simulink model "Control_Loop4_2Model"  (R2013b)
settings: Solver=ode45  StartTime=0.0  StopTime=200  RelTol=1e-3
libraries: commutil2 x756, xpclib x100, etargetslib x98, dspnetwork x98, powerlib_meascontrol x24, commcrc2 x14, dspadpt3 x4, simulink_extras x4, dspmtrx3 x4, simulink x1
(part 7 of 7)

== system Control_Loop4_2Model/GISOO-Simulation Environment/SkyMote8/Subsystem ==
  SerialData : Inport
  AM Packet type : Constant  Value=PacketType  OutDataTypeStr=double
  Bit to Integer Converter{,1..27} (28 alike) : commutil2/Bit to Integer Converter  nbits=8  bitOrder=MSB first  signedOutputValues=Unsigned  outDtype=Inherit via internal rule  outDtypeSigned=Inherit via internal rule
  Constant25 : Constant  Value=72  OutDataTypeStr=double
  Constant26 : Constant  Value=0  OutDataTypeStr=double
  Constant{27..30} (4 alike) : Constant  Value=255  OutDataTypeStr=double
  Constant31 : Constant  Value=16  OutDataTypeStr=double
  Constant32 : Constant  Value=137  OutDataTypeStr=double
  Demux1 : Demux  Outputs=28
  Demux2 : Demux  Outputs=16
  FrameByteEnd : Constant  Value=126  OutDataTypeStr=uint8
  FrameByteStart : Constant  Value=126  OutDataTypeStr=uint8
  Framing byte : Constant  Value=68  OutDataTypeStr=uint8
  General CRC Generator1 : commcrc2/General CRC Generator  genPoly=[1 0 0 0 1 0 0 0 0 0 0 1 0 0 0 0 1]  iniStates=0  directMethod=off  reflectInputBytes=off  reflectChecksums=off  finalXOR=0  numChecksums=1
  Integer to Bit Converter{,1..25} (26 alike) : commutil2/Integer to Bit Converter  nbits=8  signedInputValues=Unsigned  bitOrder=MSB first  outDtype=boolean
  Mux1 : Mux  Inputs=26
  Mux2 : Mux  Inputs=30
  SerialFrame : Outport
  wires:
  Bit to Integer Converter27/1 -> Mux2/3
  Demux1/28 -> Bit to Integer Converter27/1
  FrameByteStart/1 -> Mux2/30
  Bit to Integer Converter26/1 -> Mux2/2
  Demux1/27 -> Bit to Integer Converter26/1
  Demux1/15 -> Bit to Integer Converter18/1
  Demux1/14 -> Bit to Integer Converter13/1
  Demux1/6 -> Bit to Integer Converter5/1
  Demux1/16 -> Bit to Integer Converter19/1
  Demux1/25 -> Bit to Integer Converter22/1
  Demux1/17 -> Bit to Integer Converter14/1
  Demux1/18 -> Bit to Integer Converter15/1
  Demux1/26 -> Bit to Integer Converter23/1
  Demux1/22 -> Bit to Integer Converter25/1
  Demux1/23 -> Bit to Integer Converter20/1
  Demux1/20 -> Bit to Integer Converter17/1
  Demux1/19 -> Bit to Integer Converter16/1
  Demux1/5 -> Bit to Integer Converter4/1
  Demux1/21 -> Bit to Integer Converter24/1
  Demux1/4 -> Bit to Integer Converter3/1
  Demux1/24 -> Bit to Integer Converter21/1
  Constant31/1 -> Integer to Bit Converter7/1
  Integer to Bit Converter19/1 -> Mux1/20
  Integer to Bit Converter20/1 -> Mux1/21
  Integer to Bit Converter9/1 -> Mux1/10
  Integer to Bit Converter18/1 -> Mux1/19
  Demux1/12 -> Bit to Integer Converter11/1
  Mux2/1 -> SerialFrame/1
  Integer to Bit Converter12/1 -> Mux1/13
  Demux2/9 -> Integer to Bit Converter18/1
  Demux1/7 -> Bit to Integer Converter6/1
  Demux1/13 -> Bit to Integer Converter12/1
  Demux1/9 -> Bit to Integer Converter8/1
  Demux1/1 -> Bit to Integer Converter/1
  Demux2/11 -> Integer to Bit Converter20/1
  Demux1/11 -> Bit to Integer Converter10/1
  AM Packet type/1 -> Integer to Bit Converter9/1
  FrameByteEnd/1 -> Mux2/1
  Integer to Bit Converter22/1 -> Mux1/23
  Integer to Bit Converter21/1 -> Mux1/22
  Integer to Bit Converter25/1 -> Mux1/26
  Constant32/1 -> Integer to Bit Converter8/1
  Integer to Bit Converter8/1 -> Mux1/9
  General CRC Generator1/1 -> Demux1/1
  Integer to Bit Converter7/1 -> Mux1/8
  Demux1/3 -> Bit to Integer Converter2/1
  Integer to Bit Converter2/1 -> Mux1/3
  Integer to Bit Converter3/1 -> Mux1/4
  Constant28/1 -> Integer to Bit Converter4/1
  Integer to Bit Converter4/1 -> Mux1/5
  Constant27/1 -> Integer to Bit Converter3/1
  Constant26/1 -> Integer to Bit Converter2/1
  Constant29/1 -> Integer to Bit Converter5/1
  Integer to Bit Converter1/1 -> Mux1/2
  Integer to Bit Converter5/1 -> Mux1/6
  Demux2/14 -> Integer to Bit Converter23/1
  Demux2/16 -> Integer to Bit Converter25/1
  Mux1/1 -> General CRC Generator1/1
  Framing byte/1 -> Integer to Bit Converter/1
  Demux2/15 -> Integer to Bit Converter24/1
  Demux2/13 -> Integer to Bit Converter22/1
  Integer to Bit Converter/1 -> Mux1/1
  Demux2/12 -> Integer to Bit Converter21/1
  Constant25/1 -> Integer to Bit Converter1/1
  Demux2/8 -> Integer to Bit Converter17/1
  Integer to Bit Converter10/1 -> Mux1/11
  Demux2/10 -> Integer to Bit Converter19/1
  Integer to Bit Converter6/1 -> Mux1/7
  Demux1/2 -> Bit to Integer Converter1/1
  Integer to Bit Converter16/1 -> Mux1/17
  Integer to Bit Converter15/1 -> Mux1/16
  Integer to Bit Converter17/1 -> Mux1/18
  Integer to Bit Converter13/1 -> Mux1/14
  Demux1/8 -> Bit to Integer Converter7/1
  Demux1/10 -> Bit to Integer Converter9/1
  Constant30/1 -> Integer to Bit Converter6/1
  Integer to Bit Converter11/1 -> Mux1/12
  Integer to Bit Converter23/1 -> Mux1/24
  Integer to Bit Converter24/1 -> Mux1/25
  Integer to Bit Converter14/1 -> Mux1/15
  Demux2/6 -> Integer to Bit Converter15/1
  Demux2/5 -> Integer to Bit Converter14/1
  Bit to Integer Converter22/1 -> Mux2/5
  SerialData/1 -> Demux2/1
  Bit to Integer Converter21/1 -> Mux2/6
  Demux2/2 -> Integer to Bit Converter11/1
  Demux2/1 -> Integer to Bit Converter10/1
  Bit to Integer Converter17/1 -> Mux2/10
  Bit to Integer Converter20/1 -> Mux2/7
  Bit to Integer Converter/1 -> Mux2/29
  Bit to Integer Converter9/1 -> Mux2/20
  Bit to Integer Converter7/1 -> Mux2/22
  Bit to Integer Converter11/1 -> Mux2/18
  Bit to Integer Converter4/1 -> Mux2/25
  Bit to Integer Converter1/1 -> Mux2/28
  Bit to Integer Converter6/1 -> Mux2/23
  Bit to Integer Converter10/1 -> Mux2/19
  Bit to Integer Converter25/1 -> Mux2/8
  Bit to Integer Converter15/1 -> Mux2/12
  Bit to Integer Converter13/1 -> Mux2/16
  Bit to Integer Converter16/1 -> Mux2/11
  Bit to Integer Converter2/1 -> Mux2/27
  Bit to Integer Converter5/1 -> Mux2/24
  Demux2/7 -> Integer to Bit Converter16/1
  Bit to Integer Converter14/1 -> Mux2/13
  Bit to Integer Converter19/1 -> Mux2/14
  Bit to Integer Converter12/1 -> Mux2/17
  Bit to Integer Converter18/1 -> Mux2/15
  Demux2/3 -> Integer to Bit Converter12/1
  Bit to Integer Converter8/1 -> Mux2/21
  Bit to Integer Converter24/1 -> Mux2/9
  Demux2/4 -> Integer to Bit Converter13/1
  Bit to Integer Converter3/1 -> Mux2/26
  Bit to Integer Converter23/1 -> Mux2/4

== system Control_Loop4_2Model/GISOO-Simulation Environment/SkyMote8/Triggered Subsystem ==
  In2 : Inport
  Trigger : TriggerPort
  Byte Reversal1 : etargetslib/Byte Reversal  numInp=1
  Data Type Conversion1 : DataTypeConversion  OutDataTypeStr=uint32
  Pack : xpclib/UDP/Pack  datatypes={'uint32'}  byteAlign=1
  UDP Send : dspnetwork/UDP Send  remoteURL='127.0.0.1'  remotePort=18000+moteID  localURL='0.0.0.0'  localPortSource=Automatically determine  localPort=-1  sampletime=-1  separateLengthPort=0
  wires:
  Data Type Conversion1/1 -> Byte Reversal1/1
  Byte Reversal1/1 -> Pack/1
  Pack/1 -> UDP Send/1
  In2/1 -> Data Type Conversion1/1

== system Control_Loop4_2Model/GISOO-Simulation Environment/SkyMote8/Triggered Subsystem1 ==
  In2 : Inport
  Trigger : TriggerPort
  Byte Reversal1 : etargetslib/Byte Reversal  numInp=1
  Data Type Conversion1 : DataTypeConversion  OutDataTypeStr=uint32
  Pack : xpclib/UDP/Pack  datatypes={'uint32'}  byteAlign=1
  UDP Send : dspnetwork/UDP Send  remoteURL='127.0.0.1'  remotePort=18000+moteID  localURL='0.0.0.0'  localPortSource=Automatically determine  localPort=-1  sampletime=-1  separateLengthPort=0
  wires:
  Byte Reversal1/1 -> Pack/1
  Data Type Conversion1/1 -> Byte Reversal1/1
  In2/1 -> Data Type Conversion1/1
  Pack/1 -> UDP Send/1

== system Control_Loop4_2Model/GISOO-Simulation Environment/SkyMote8/Triggered Subsystem2 ==
  In2 : Inport
  Trigger : TriggerPort
  Byte Reversal : etargetslib/Byte Reversal  numInp=1
  Data Type Conversion1 : DataTypeConversion  OutDataTypeStr=uint32
  Pack : xpclib/UDP/Pack  datatypes={'uint32'}  byteAlign=1
  UDP Send : dspnetwork/UDP Send  remoteURL='127.0.0.1'  remotePort=18000+moteID  localURL='0.0.0.0'  localPortSource=Automatically determine  localPort=-1  sampletime=-1  separateLengthPort=0
  Out1 : Outport
  wires:
  Byte Reversal/1 -> Pack/1
  Pack/1 -> UDP Send/1
  Data Type Conversion1/1 -> Byte Reversal/1, Out1/1
  In2/1 -> Data Type Conversion1/1

== system Control_Loop4_2Model/GISOO-Simulation Environment/SkyMote8/Triggered Subsystem3 ==
  In2 : Inport
  Trigger : TriggerPort
  Byte Reversal : etargetslib/Byte Reversal  numInp=1
  Data Type Conversion1 : DataTypeConversion  OutDataTypeStr=uint32
  Pack : xpclib/UDP/Pack  datatypes={'uint32'}  byteAlign=1
  UDP Send : dspnetwork/UDP Send  remoteURL='127.0.0.1'  remotePort=18000+moteID  localURL='0.0.0.0'  localPortSource=Automatically determine  localPort=-1  sampletime=-1  separateLengthPort=0
  Out1 : Outport
  wires:
  Byte Reversal/1 -> Pack/1
  In2/1 -> Data Type Conversion1/1
  Data Type Conversion1/1 -> Out1/1, Byte Reversal/1
  Pack/1 -> UDP Send/1

== system Control_Loop4_2Model/GISOO-Simulation Environment/SkyMote8/Triggered Subsystem4 ==
  RecivedSD : Inport
  Trigger : TriggerPort
  Byte Reversal : etargetslib/Byte Reversal  numInp=1
  Constant : Constant  Value=1111
  Data Type Conversion1 : DataTypeConversion  OutDataTypeStr=uint32
  Pack : xpclib/UDP/Pack  datatypes={'uint32'}  byteAlign=1
  UDP Send : dspnetwork/UDP Send  remoteURL='127.0.0.1'  remotePort=18000+moteID  localURL='0.0.0.0'  localPortSource=Automatically determine  localPort=-1  sampletime=-1  separateLengthPort=0
  SDToApplay : Outport
  wires:
  Data Type Conversion1/1 -> Byte Reversal/1
  Byte Reversal/1 -> Pack/1
  Constant/1 -> Data Type Conversion1/1
  RecivedSD/1 -> SDToApplay/1
  Pack/1 -> UDP Send/1

== system Control_Loop4_2Model/GISOO-Simulation Environment/SkyMote8/Triggered Subsystem5 ==
  SerialDataToSend : Inport
  Trigger : TriggerPort
  Byte Reversal : etargetslib/Byte Reversal  numInp=1
  Demux : Demux  Outputs=30
  Pack : xpclib/UDP/Pack  datatypes={'uint8','uint8','uint8','uint8','uint8','uint8','uint8','uint8','uint8','uint8','uint8','uint8','uint8','uint8','uint8','uint8','uint8','uint8','uint8','uint8','uint8','uint8','uint8','uint8','uint8','uint8','uint8','uint8','uint8','uint8'}  byteAlign=1
  UDP Send : dspnetwork/UDP Send  remoteURL='127.0.0.1'  remotePort=18000+moteID  localURL='0.0.0.0'  localPortSource=Automatically determine  localPort=-1  sampletime=-1  separateLengthPort=0
  wires:
  Pack/1 -> UDP Send/1
  Demux/1 -> Pack/1
  Demux/2 -> Pack/2
  Demux/3 -> Pack/3
  Demux/4 -> Pack/4
  Demux/5 -> Pack/5
  Demux/6 -> Pack/6
  Demux/7 -> Pack/7
  Demux/8 -> Pack/8
  Demux/9 -> Pack/9
  Demux/10 -> Pack/10
  Demux/11 -> Pack/11
  Demux/12 -> Pack/12
  Demux/13 -> Pack/13
  Demux/14 -> Pack/14
  Demux/15 -> Pack/15
  Demux/16 -> Pack/16
  Demux/17 -> Pack/17
  Demux/18 -> Pack/18
  Demux/19 -> Pack/19
  Demux/20 -> Pack/20
  Demux/21 -> Pack/21
  Demux/22 -> Pack/22
  Demux/23 -> Pack/23
  Demux/24 -> Pack/24
  Demux/25 -> Pack/25
  Demux/26 -> Pack/26
  Demux/27 -> Pack/27
  Demux/28 -> Pack/28
  Demux/29 -> Pack/29
  Demux/30 -> Pack/30
  SerialDataToSend/1 -> Byte Reversal/1
  Byte Reversal/1 -> Demux/1

== system Control_Loop4_2Model/GISOO-Simulation Environment/SkyMote9/ADC0 Sender ==
  In2 : Inport
  Trigger : TriggerPort
  Byte Reversal1 : etargetslib/Byte Reversal  numInp=1
  Data Type Conversion1 : DataTypeConversion  OutDataTypeStr=uint32
  Pack : xpclib/UDP/Pack  datatypes={'uint32'}  byteAlign=1
  UDP Send : dspnetwork/UDP Send  remoteURL='127.0.0.1'  remotePort=18000+moteID  localURL='0.0.0.0'  localPortSource=Automatically determine  localPort=-1  sampletime=-1  separateLengthPort=0
  wires:
  Data Type Conversion1/1 -> Byte Reversal1/1
  Byte Reversal1/1 -> Pack/1
  In2/1 -> Data Type Conversion1/1
  Pack/1 -> UDP Send/1

== system Control_Loop4_2Model/GISOO-Simulation Environment/SkyMote9/Subsystem ==
  SerialData : Inport
  AM Packet type : Constant  Value=PacketType  OutDataTypeStr=double
  Bit to Integer Converter{,1..27} (28 alike) : commutil2/Bit to Integer Converter  nbits=8  bitOrder=MSB first  signedOutputValues=Unsigned  outDtype=Inherit via internal rule  outDtypeSigned=Inherit via internal rule
  Constant25 : Constant  Value=72  OutDataTypeStr=double
  Constant26 : Constant  Value=0  OutDataTypeStr=double
  Constant{27..30} (4 alike) : Constant  Value=255  OutDataTypeStr=double
  Constant31 : Constant  Value=16  OutDataTypeStr=double
  Constant32 : Constant  Value=137  OutDataTypeStr=double
  Demux1 : Demux  Outputs=28
  Demux2 : Demux  Outputs=16
  FrameByteEnd : Constant  Value=126  OutDataTypeStr=uint8
  FrameByteStart : Constant  Value=126  OutDataTypeStr=uint8
  Framing byte : Constant  Value=68  OutDataTypeStr=uint8
  General CRC Generator1 : commcrc2/General CRC Generator  genPoly=[1 0 0 0 1 0 0 0 0 0 0 1 0 0 0 0 1]  iniStates=0  directMethod=off  reflectInputBytes=off  reflectChecksums=off  finalXOR=0  numChecksums=1
  Integer to Bit Converter{,1..25} (26 alike) : commutil2/Integer to Bit Converter  nbits=8  signedInputValues=Unsigned  bitOrder=MSB first  outDtype=boolean
  Mux1 : Mux  Inputs=26
  Mux2 : Mux  Inputs=30
  SerialFrame : Outport
  wires:
  Bit to Integer Converter27/1 -> Mux2/3
  Demux1/28 -> Bit to Integer Converter27/1
  FrameByteStart/1 -> Mux2/30
  Bit to Integer Converter26/1 -> Mux2/2
  Demux1/27 -> Bit to Integer Converter26/1
  Demux1/15 -> Bit to Integer Converter18/1
  Demux1/14 -> Bit to Integer Converter13/1
  Demux1/6 -> Bit to Integer Converter5/1
  Demux1/16 -> Bit to Integer Converter19/1
  Demux1/25 -> Bit to Integer Converter22/1
  Demux1/17 -> Bit to Integer Converter14/1
  Demux1/18 -> Bit to Integer Converter15/1
  Demux1/26 -> Bit to Integer Converter23/1
  Demux1/22 -> Bit to Integer Converter25/1
  Demux1/23 -> Bit to Integer Converter20/1
  Demux1/20 -> Bit to Integer Converter17/1
  Demux1/19 -> Bit to Integer Converter16/1
  Demux1/5 -> Bit to Integer Converter4/1
  Demux1/21 -> Bit to Integer Converter24/1
  Demux1/4 -> Bit to Integer Converter3/1
  Demux1/24 -> Bit to Integer Converter21/1
  Constant31/1 -> Integer to Bit Converter7/1
  Integer to Bit Converter19/1 -> Mux1/20
  Integer to Bit Converter20/1 -> Mux1/21
  Integer to Bit Converter9/1 -> Mux1/10
  Integer to Bit Converter18/1 -> Mux1/19
  Demux1/12 -> Bit to Integer Converter11/1
  Mux2/1 -> SerialFrame/1
  Integer to Bit Converter12/1 -> Mux1/13
  Demux2/9 -> Integer to Bit Converter18/1
  Demux1/7 -> Bit to Integer Converter6/1
  Demux1/13 -> Bit to Integer Converter12/1
  Demux1/9 -> Bit to Integer Converter8/1
  Demux1/1 -> Bit to Integer Converter/1
  Demux2/11 -> Integer to Bit Converter20/1
  Demux1/11 -> Bit to Integer Converter10/1
  AM Packet type/1 -> Integer to Bit Converter9/1
  FrameByteEnd/1 -> Mux2/1
  Integer to Bit Converter22/1 -> Mux1/23
  Integer to Bit Converter21/1 -> Mux1/22
  Integer to Bit Converter25/1 -> Mux1/26
  Constant32/1 -> Integer to Bit Converter8/1
  Integer to Bit Converter8/1 -> Mux1/9
  General CRC Generator1/1 -> Demux1/1
  Integer to Bit Converter7/1 -> Mux1/8
  Demux1/3 -> Bit to Integer Converter2/1
  Integer to Bit Converter2/1 -> Mux1/3
  Integer to Bit Converter3/1 -> Mux1/4
  Constant28/1 -> Integer to Bit Converter4/1
  Integer to Bit Converter4/1 -> Mux1/5
  Constant27/1 -> Integer to Bit Converter3/1
  Constant26/1 -> Integer to Bit Converter2/1
  Constant29/1 -> Integer to Bit Converter5/1
  Integer to Bit Converter1/1 -> Mux1/2
  Integer to Bit Converter5/1 -> Mux1/6
  Demux2/14 -> Integer to Bit Converter23/1
  Demux2/16 -> Integer to Bit Converter25/1
  Mux1/1 -> General CRC Generator1/1
  Framing byte/1 -> Integer to Bit Converter/1
  Demux2/15 -> Integer to Bit Converter24/1
  Demux2/13 -> Integer to Bit Converter22/1
  Integer to Bit Converter/1 -> Mux1/1
  Demux2/12 -> Integer to Bit Converter21/1
  Constant25/1 -> Integer to Bit Converter1/1
  Demux2/8 -> Integer to Bit Converter17/1
  Integer to Bit Converter10/1 -> Mux1/11
  Demux2/10 -> Integer to Bit Converter19/1
  Integer to Bit Converter6/1 -> Mux1/7
  Demux1/2 -> Bit to Integer Converter1/1
  Integer to Bit Converter16/1 -> Mux1/17
  Integer to Bit Converter15/1 -> Mux1/16
  Integer to Bit Converter17/1 -> Mux1/18
  Integer to Bit Converter13/1 -> Mux1/14
  Demux1/8 -> Bit to Integer Converter7/1
  Demux1/10 -> Bit to Integer Converter9/1
  Constant30/1 -> Integer to Bit Converter6/1
  Integer to Bit Converter11/1 -> Mux1/12
  Integer to Bit Converter23/1 -> Mux1/24
  Integer to Bit Converter24/1 -> Mux1/25
  Integer to Bit Converter14/1 -> Mux1/15
  Demux2/6 -> Integer to Bit Converter15/1
  Demux2/5 -> Integer to Bit Converter14/1
  Bit to Integer Converter22/1 -> Mux2/5
  SerialData/1 -> Demux2/1
  Bit to Integer Converter21/1 -> Mux2/6
  Demux2/2 -> Integer to Bit Converter11/1
  Demux2/1 -> Integer to Bit Converter10/1
  Bit to Integer Converter17/1 -> Mux2/10
  Bit to Integer Converter20/1 -> Mux2/7
  Bit to Integer Converter/1 -> Mux2/29
  Bit to Integer Converter9/1 -> Mux2/20
  Bit to Integer Converter7/1 -> Mux2/22
  Bit to Integer Converter11/1 -> Mux2/18
  Bit to Integer Converter4/1 -> Mux2/25
  Bit to Integer Converter1/1 -> Mux2/28
  Bit to Integer Converter6/1 -> Mux2/23
  Bit to Integer Converter10/1 -> Mux2/19
  Bit to Integer Converter25/1 -> Mux2/8
  Bit to Integer Converter15/1 -> Mux2/12
  Bit to Integer Converter13/1 -> Mux2/16
  Bit to Integer Converter16/1 -> Mux2/11
  Bit to Integer Converter2/1 -> Mux2/27
  Bit to Integer Converter5/1 -> Mux2/24
  Demux2/7 -> Integer to Bit Converter16/1
  Bit to Integer Converter14/1 -> Mux2/13
  Bit to Integer Converter19/1 -> Mux2/14
  Bit to Integer Converter12/1 -> Mux2/17
  Bit to Integer Converter18/1 -> Mux2/15
  Demux2/3 -> Integer to Bit Converter12/1
  Bit to Integer Converter8/1 -> Mux2/21
  Bit to Integer Converter24/1 -> Mux2/9
  Demux2/4 -> Integer to Bit Converter13/1
  Bit to Integer Converter3/1 -> Mux2/26
  Bit to Integer Converter23/1 -> Mux2/4

== system Control_Loop4_2Model/GISOO-Simulation Environment/SkyMote9/Triggered Subsystem ==
  In2 : Inport
  Trigger : TriggerPort
  Byte Reversal1 : etargetslib/Byte Reversal  numInp=1
  Data Type Conversion1 : DataTypeConversion  OutDataTypeStr=uint32
  Pack : xpclib/UDP/Pack  datatypes={'uint32'}  byteAlign=1
  UDP Send : dspnetwork/UDP Send  remoteURL='127.0.0.1'  remotePort=18000+moteID  localURL='0.0.0.0'  localPortSource=Automatically determine  localPort=-1  sampletime=-1  separateLengthPort=0
  wires:
  Data Type Conversion1/1 -> Byte Reversal1/1
  Byte Reversal1/1 -> Pack/1
  Pack/1 -> UDP Send/1
  In2/1 -> Data Type Conversion1/1

== system Control_Loop4_2Model/GISOO-Simulation Environment/SkyMote9/Triggered Subsystem1 ==
  In2 : Inport
  Trigger : TriggerPort
  Byte Reversal1 : etargetslib/Byte Reversal  numInp=1
  Data Type Conversion1 : DataTypeConversion  OutDataTypeStr=uint32
  Pack : xpclib/UDP/Pack  datatypes={'uint32'}  byteAlign=1
  UDP Send : dspnetwork/UDP Send  remoteURL='127.0.0.1'  remotePort=18000+moteID  localURL='0.0.0.0'  localPortSource=Automatically determine  localPort=-1  sampletime=-1  separateLengthPort=0
  wires:
  Byte Reversal1/1 -> Pack/1
  Data Type Conversion1/1 -> Byte Reversal1/1
  In2/1 -> Data Type Conversion1/1
  Pack/1 -> UDP Send/1

== system Control_Loop4_2Model/GISOO-Simulation Environment/SkyMote9/Triggered Subsystem2 ==
  In2 : Inport
  Trigger : TriggerPort
  Byte Reversal : etargetslib/Byte Reversal  numInp=1
  Data Type Conversion1 : DataTypeConversion  OutDataTypeStr=uint32
  Pack : xpclib/UDP/Pack  datatypes={'uint32'}  byteAlign=1
  UDP Send : dspnetwork/UDP Send  remoteURL='127.0.0.1'  remotePort=18000+moteID  localURL='0.0.0.0'  localPortSource=Automatically determine  localPort=-1  sampletime=-1  separateLengthPort=0
  Out1 : Outport
  wires:
  Byte Reversal/1 -> Pack/1
  Pack/1 -> UDP Send/1
  Data Type Conversion1/1 -> Byte Reversal/1, Out1/1
  In2/1 -> Data Type Conversion1/1

== system Control_Loop4_2Model/GISOO-Simulation Environment/SkyMote9/Triggered Subsystem3 ==
  In2 : Inport
  Trigger : TriggerPort
  Byte Reversal : etargetslib/Byte Reversal  numInp=1
  Data Type Conversion1 : DataTypeConversion  OutDataTypeStr=uint32
  Pack : xpclib/UDP/Pack  datatypes={'uint32'}  byteAlign=1
  UDP Send : dspnetwork/UDP Send  remoteURL='127.0.0.1'  remotePort=18000+moteID  localURL='0.0.0.0'  localPortSource=Automatically determine  localPort=-1  sampletime=-1  separateLengthPort=0
  Out1 : Outport
  wires:
  Byte Reversal/1 -> Pack/1
  In2/1 -> Data Type Conversion1/1
  Data Type Conversion1/1 -> Out1/1, Byte Reversal/1
  Pack/1 -> UDP Send/1

== system Control_Loop4_2Model/GISOO-Simulation Environment/SkyMote9/Triggered Subsystem4 ==
  RecivedSD : Inport
  Trigger : TriggerPort
  Byte Reversal : etargetslib/Byte Reversal  numInp=1
  Constant : Constant  Value=1111
  Data Type Conversion1 : DataTypeConversion  OutDataTypeStr=uint32
  Pack : xpclib/UDP/Pack  datatypes={'uint32'}  byteAlign=1
  UDP Send : dspnetwork/UDP Send  remoteURL='127.0.0.1'  remotePort=18000+moteID  localURL='0.0.0.0'  localPortSource=Automatically determine  localPort=-1  sampletime=-1  separateLengthPort=0
  SDToApplay : Outport
  wires:
  Data Type Conversion1/1 -> Byte Reversal/1
  Byte Reversal/1 -> Pack/1
  Constant/1 -> Data Type Conversion1/1
  RecivedSD/1 -> SDToApplay/1
  Pack/1 -> UDP Send/1

== system Control_Loop4_2Model/GISOO-Simulation Environment/SkyMote9/Triggered Subsystem5 ==
  SerialDataToSend : Inport
  Trigger : TriggerPort
  Byte Reversal : etargetslib/Byte Reversal  numInp=1
  Demux : Demux  Outputs=30
  Pack : xpclib/UDP/Pack  datatypes={'uint8','uint8','uint8','uint8','uint8','uint8','uint8','uint8','uint8','uint8','uint8','uint8','uint8','uint8','uint8','uint8','uint8','uint8','uint8','uint8','uint8','uint8','uint8','uint8','uint8','uint8','uint8','uint8','uint8','uint8'}  byteAlign=1
  UDP Send : dspnetwork/UDP Send  remoteURL='127.0.0.1'  remotePort=18000+moteID  localURL='0.0.0.0'  localPortSource=Automatically determine  localPort=-1  sampletime=-1  separateLengthPort=0
  wires:
  Pack/1 -> UDP Send/1
  Demux/1 -> Pack/1
  Demux/2 -> Pack/2
  Demux/3 -> Pack/3
  Demux/4 -> Pack/4
  Demux/5 -> Pack/5
  Demux/6 -> Pack/6
  Demux/7 -> Pack/7
  Demux/8 -> Pack/8
  Demux/9 -> Pack/9
  Demux/10 -> Pack/10
  Demux/11 -> Pack/11
  Demux/12 -> Pack/12
  Demux/13 -> Pack/13
  Demux/14 -> Pack/14
  Demux/15 -> Pack/15
  Demux/16 -> Pack/16
  Demux/17 -> Pack/17
  Demux/18 -> Pack/18
  Demux/19 -> Pack/19
  Demux/20 -> Pack/20
  Demux/21 -> Pack/21
  Demux/22 -> Pack/22
  Demux/23 -> Pack/23
  Demux/24 -> Pack/24
  Demux/25 -> Pack/25
  Demux/26 -> Pack/26
  Demux/27 -> Pack/27
  Demux/28 -> Pack/28
  Demux/29 -> Pack/29
  Demux/30 -> Pack/30
  SerialDataToSend/1 -> Byte Reversal/1
  Byte Reversal/1 -> Demux/1

== matlab function Control_Loop4_2Model/extractdec_F2/ChangeVal ==
  data: u input; y1 output; y2 output
function [y1,y2]= fcn(u)
y1 = 0;
y2 = 0;
%#codegen
if (u >= 0)
    temp1 = floor(u);
    temp2 = (u - floor(u))*1000;
    y1 = temp1;
    %Fid
    y2 = temp2+1000;
    %y1 = dec2bin(y1);
    %y2 = dec2bin(y2);
elseif (u < 0)
    temp2 = (ceil(u) - u)*(1000);
    temp2 = abs(floor(temp2));
    %-ve values
    temp1 = abs(ceil(u)) + 1000;
    y1 = temp1;
    %Fid
    y2 = temp2+1000;
    %y1 = dec2bin(y1);
    %y1 = bitor(y1,2048);
    %y2 = dec2bin(y2);
end
end

== matlab function Control_Loop4_2Model/extractdec_F3/ChangeVal ==
  data: u input; y1 output; y2 output
function [y1,y2]= fcn(u)
y1 = 0;
y2 = 0;
%#codegen
if (u >= 0)
    temp1 = floor(u);
    temp2 = (u - floor(u))*1000;
    y1 = temp1;
    %Fid
    y2 = temp2+2000;
    %y1 = dec2bin(y1);
    %y2 = dec2bin(y2);
elseif (u < 0)
    temp2 = (ceil(u) - u)*(1000);
    temp2 = abs(floor(temp2));
    %-ve values
    temp1 = abs(ceil(u)) + 1000;
    y1 = temp1;
    %Fid
    y2 = temp2+2000;
    %y1 = dec2bin(y1);
    %y1 = bitor(y1,2048);
    %y2 = dec2bin(y2);
end
end

== matlab function Control_Loop4_2Model/extractdec_F4/ChangeVal ==
  data: u input; y1 output; y2 output
function [y1,y2]= fcn(u)
y1 = 0;
y2 = 0;
%#codegen
if (u >= 0)
    temp1 = floor(u);
    temp2 = (u - floor(u))*1000;
    y1 = temp1;
    y2 = temp2+3000;
    %y1 = dec2bin(y1);
    %y2 = dec2bin(y2);
elseif (u < 0)
    temp2 = (ceil(u) - u)*(1000);
    temp2 = abs(floor(temp2));
    temp1 = abs(ceil(u)) + 1000;
    y1 = temp1;
    y2 = temp2+3000;
    %y1 = dec2bin(y1);
    %y1 = bitor(y1,2048);
    %y2 = dec2bin(y2);
end
end

== matlab function Control_Loop4_2Model/Decimal1/combineDecimal_1 ==
  data: u1 input; u2 input; y1 output; y2 output; y3 output; y4 output; x1 output; x2 output; x3 output; x4 output; x1_prev input; x2_prev input; x3_prev input; x4_prev input
function [y1,y2,y3,y4,x1,x2,x3,x4] = fcn(u1,u2,x1_prev,x2_prev,x3_prev,x4_prev)


%#codegen
if (u1 >= 1000)
    u1 = u1 - 1000;
    if (u2 >= 3000)
        u2 = u2 - 3000;
        y4 = - (u1 + u2*0.001);
        y3 = x3_prev;
        y2 = x2_prev;
        y1 = x1_prev;
    elseif (u2 < 3000 && u2 >= 2000)
        u2 = u2 - 2000;
        y4 = x4_prev;
        y3 = - (u1 + u2*0.001);
        y2 = x2_prev;
        y1 = x1_prev;
    elseif (u2 < 2000 && u2 >= 1000)
        u2 = u2 - 1000;
        y4 = x4_prev;
        y3 = x3_prev;
        y2 = - (u1 + u2*0.001);
        y1 = x1_prev;
    else
        y4 = x4_prev;
        y3 = x3_prev;
        y2 = x2_prev;
        y1 = - (u1 + u2*0.001);
    end
else
    if (u2 >= 3000)
        u2 = u2 - 3000;
        y4 = (u1 + u2*0.001);
        y3 = x3_prev;
        y2 = x2_prev;
        y1 = x1_prev;
    elseif (u2 < 3000 && u2 >= 2000)
        u2 = u2 - 2000;
        y4 = x4_prev;
        y3 = (u1 + u2*0.001);
        y2 = x2_prev;
        y1 = x1_prev;
    elseif (u2 < 2000 && u2 >= 1000)
        u2 = u2 - 1000;
        y4 = x4_prev;
        y3 = x3_prev;
        y2 = (u1 + u2*0.001);
        y1 = x1_prev;
    else
        y4 = x4_prev;
        y3 = x3_prev;
        y2 = x2_prev;
        y1 = (u1 + u2*0.001);
    end
end
x4 = y4;
x3 = y3;
x2 = y2;
x1 = y1;
end

== matlab function Control_Loop4_2Model/extractdec_F5/ChangeVal ==
  data: u1 input; y1 output; y2 output; u2 input; u3 input; u4 input; counter data_store_memory
function [y1,y2] = fcn(u1,u2,u3,u4)
global counter;
y1 = 0;
y2 = 0;
if (mod(counter,4) == 0)
    if (u1 >= 0)
        temp1 = floor(u1);
        temp2 = (u1 - floor(u1))*1000;
        y1 = temp1;
        y2 = temp2;
    elseif (u1 < 0)
        temp2 = (ceil(u1) - u1)*(1000);
        %-ve values
        temp2 = abs(floor(temp2));
        %Fid
        temp1 = abs(ceil(u1)) + 1000;
        y1 = temp1;
        y2 = temp2;
    end
    counter = counter + 1;
elseif (mod(counter,4) == 1)
    if (u2 >= 0)
        temp1 = floor(u2);
        temp2 = (u2 - floor(u2))*1000;
        y1 = temp1;
        y2 = temp2+1000;
    elseif (u2 < 0)
        temp2 = (ceil(u2) - u2)*(1000);
        %-ve values
        temp2 = abs(floor(temp2));
        %Fid
        temp1 = abs(ceil(u2));
        y1 = temp1+1000;
        y2 = temp2+1000;
    end
    counter = counter + 1;
elseif (mod(counter,4) == 2)
    if (u3 >= 0)
        temp1 = floor(u3);
        temp2 = (u3 - floor(u3))*1000;
        y1 = temp1;
        y2 = temp2+2000;
    elseif (u3 < 0)
        temp2 = (ceil(u3) - u3)*(1000);
        %-ve values
        temp2 = abs(floor(temp2));
        %Fid
        temp1 = abs(ceil(u3));
        y1 = temp1+1000;
        y2 = temp2+2000;
    end
    counter = counter + 1;
elseif (mod(counter,4) == 3)
    if (u4 >= 0)
        temp1 = floor(u4);
        temp2 = (u4 - floor(u4))*1000;
        y1 = temp1;
        y2 = temp2+3000;
    elseif (u4 < 0)
        temp2 = (ceil(u4) - u4)*(1000);
        %-ve values
        temp2 = abs(floor(temp2));
        %Fid
        temp1 = abs(ceil(u4));
        y1 = temp1+1000;
        y2 = temp2+3000;
    end
    counter = counter - 3;
end
end

== matlab function Control_Loop4_2Model/Decimal2/combineDecimal_1 ==
  data: u1 input; u2 input; y output
function y = fcn(u1,u2)


%#codegen
if (u1 >= 1000)
    u1 = u1 - 1000;
    %if (u2 >= 1000)
     %   u2 = u2 - 1000;
        y = - (u1 + u2*0.001);
        %y2 = y;
        %y1 = u1_prev;
    %else
     %   y = - (u1 + u2*0.001);
     %   y1 = y;
     %   y2 = u2_prev;
    %end
else
    %if (u2 >= 1000)
    %    u2 = u2 - 1000;
        y = (u1 + u2*0.001);
     %   y2 = y;
     %   y1 = u1_prev;
    %else
     %   y = (u1 + u2*0.001);
     %   y1 = y;
     %   y2 = u2_prev;
    %end
end
%x = y;
%x2 = y2;
%if (u1 > 2047)
%    u1 = -(4096 - u1);
%    u2 = u2 * (-0.01);
%else
%    u2 = u2 * (0.01);
%end
%y = u1 + u2;
%if y == 0.00
%    if x == 0.00
%        y = 0.00;
%    end
%end
%x1 = y;
%if u > 2047
  %  u = -(4096 - u);
%end
%u = u * 0.1;
%if u > 0.0
 %   y = u;
%elseif u < 0.0
%    y = u;
%else
%    y = x;
%end  
%if (u > 3095)
%    u = -(4096 - u)/10;
%else
%    u = u/10;
%end
%y = u;
%u = u/10 - 100;
%if (u > 0.0)
%    y = u;
%elseif (u < 0.0)
%    y = u;
%else
%if u == 0
%    y = x;
%else
%    y = u;
%end
end

== matlab function Control_Loop4_2Model/Decimal3/combineDecimal_1 ==
  data: u1 input; u2 input; y output
function y = fcn(u1,u2)

u2 = u2 - 1000;
%#codegen
if (u1 >= 1000)
    u1 = u1 - 1000;
    %if (u2 >= 1000)
     %   u2 = u2 - 1000;
        y = - (u1 + u2*0.001);
        %y2 = y;
        %y1 = u1_prev;
    %else
     %   y = - (u1 + u2*0.001);
     %   y1 = y;
     %   y2 = u2_prev;
    %end
else
    %if (u2 >= 1000)
    %    u2 = u2 - 1000;
        y = (u1 + u2*0.001);
     %   y2 = y;
     %   y1 = u1_prev;
    %else
     %   y = (u1 + u2*0.001);
     %   y1 = y;
     %   y2 = u2_prev;
    %end
end
%x = y;
%x2 = y2;
%if (u1 > 2047)
%    u1 = -(4096 - u1);
%    u2 = u2 * (-0.01);
%else
%    u2 = u2 * (0.01);
%end
%y = u1 + u2;
%if y == 0.00
%    if x == 0.00
%        y = 0.00;
%    end
%end
%x1 = y;
%if u > 2047
  %  u = -(4096 - u);
%end
%u = u * 0.1;
%if u > 0.0
 %   y = u;
%elseif u < 0.0
%    y = u;
%else
%    y = x;
%end  
%if (u > 3095)
%    u = -(4096 - u)/10;
%else
%    u = u/10;
%end
%y = u;
%u = u/10 - 100;
%if (u > 0.0)
%    y = u;
%elseif (u < 0.0)
%    y = u;
%else
%if u == 0
%    y = x;
%else
%    y = u;
%end
end

== matlab function Control_Loop4_2Model/Decimal4/combineDecimal_1 ==
  data: u1 input; u2 input; y output
function y = fcn(u1,u2)

u2 = u2 - 2000;
%#codegen
if (u1 >= 1000)
    u1 = u1 - 1000;
    %if (u2 >= 1000)
     %   u2 = u2 - 1000;
        y = - (u1 + u2*0.001);
        %y2 = y;
        %y1 = u1_prev;
    %else
     %   y = - (u1 + u2*0.001);
     %   y1 = y;
     %   y2 = u2_prev;
    %end
else
    %if (u2 >= 1000)
    %    u2 = u2 - 1000;
        y = (u1 + u2*0.001);
     %   y2 = y;
     %   y1 = u1_prev;
    %else
     %   y = (u1 + u2*0.001);
     %   y1 = y;
     %   y2 = u2_prev;
    %end
end
%x = y;
%x2 = y2;
%if (u1 > 2047)
%    u1 = -(4096 - u1);
%    u2 = u2 * (-0.01);
%else
%    u2 = u2 * (0.01);
%end
%y = u1 + u2;
%if y == 0.00
%    if x == 0.00
%        y = 0.00;
%    end
%end
%x1 = y;
%if u > 2047
  %  u = -(4096 - u);
%end
%u = u * 0.1;
%if u > 0.0
 %   y = u;
%elseif u < 0.0
%    y = u;
%else
%    y = x;
%end  
%if (u > 3095)
%    u = -(4096 - u)/10;
%else
%    u = u/10;
%end
%y = u;
%u = u/10 - 100;
%if (u > 0.0)
%    y = u;
%elseif (u < 0.0)
%    y = u;
%else
%if u == 0
%    y = x;
%else
%    y = u;
%end
end

== matlab function Control_Loop4_2Model/Decimal5/combineDecimal_1 ==
  data: u1 input; u2 input; y output
function y = fcn(u1,u2)

u2 = u2 - 3000;
%#codegen
if (u1 >= 1000)
    u1 = u1 - 1000;
    %if (u2 >= 1000)
     %   u2 = u2 - 1000;
        y = - (u1 + u2*0.001);
        %y2 = y;
        %y1 = u1_prev;
    %else
     %   y = - (u1 + u2*0.001);
     %   y1 = y;
     %   y2 = u2_prev;
    %end
else
    %if (u2 >= 1000)
    %    u2 = u2 - 1000;
        y = (u1 + u2*0.001);
     %   y2 = y;
     %   y1 = u1_prev;
    %else
     %   y = (u1 + u2*0.001);
     %   y1 = y;
     %   y2 = u2_prev;
    %end
end
%x = y;
%x2 = y2;
%if (u1 > 2047)
%    u1 = -(4096 - u1);
%    u2 = u2 * (-0.01);
%else
%    u2 = u2 * (0.01);
%end
%y = u1 + u2;
%if y == 0.00
%    if x == 0.00
%        y = 0.00;
%    end
%end
%x1 = y;
%if u > 2047
  %  u = -(4096 - u);
%end
%u = u * 0.1;
%if u > 0.0
 %   y = u;
%elseif u < 0.0
%    y = u;
%else
%    y = x;
%end  
%if (u > 3095)
%    u = -(4096 - u)/10;
%else
%    u = u/10;
%end
%y = u;
%u = u/10 - 100;
%if (u > 0.0)
%    y = u;
%elseif (u < 0.0)
%    y = u;
%else
%if u == 0
%    y = x;
%else
%    y = u;
%end
end

== matlab function Control_Loop4_2Model/extractdec_F1/ChangeVal ==
  data: u input; y1 output; y2 output
function [y1,y2]= fcn(u)
y1 = 0;
y2 = 0;
%#codegen
if (u >= 0)
    temp1 = floor(u);
    temp2 = (u - floor(u))*1000;
    y1 = temp1;
    y2 = temp2;
    %y1 = dec2bin(y1);
    %y2 = dec2bin(y2);
elseif (u < 0)
    temp2 = (ceil(u) - u)*(1000);
    temp2 = abs(floor(temp2));
    %-ve values
    temp1 = abs(ceil(u)) + 1000;
    y1 = temp1;
    y2 = temp2;
    %y1 = dec2bin(y1);
    %y1 = bitor(y1,2048);
    %y2 = dec2bin(y2);
end
end

== matlab function Control_Loop4_2Model/PeriodAdaptation_2 ==
  data: timer input; Vxt input; y output; period_index_2 data_store_memory; t0 input; t1 output; Vxt0_1 input; Vxt0 output; current_period_2 data_store_memory; tau_2 data_store_memory; last_adaptation_2 data_store_memory
function [y,t1,Vxt0]= fcn(timer,Vxt,t0,Vxt0_1)
%#codegen
global current_period_2;
global period_index_2;
global tau_2;
global last_adaptation_2;

t1 = 0;
candidate_period = [10,20,60];   
no_of_candidates = 3;
alpha_1 = -31.4772;
alpha_2 = 3.7059;
beta = 1;
X_SE2 = 0.01;
Lambda = 0.1;
Vlth = alpha_1*X_SE2;
Vdth = Vlth * Lambda;

%disp(Vxt);
%disp(Vdth);
if (Vxt < Vdth)
    tau_2 = tau_2 + 1; 
    %disp(tau_1);
    if (tau_2 == 100)
        if (current_period_2 < candidate_period(no_of_candidates))
            current_period_2 = candidate_period(period_index_2 + 1);
            period_index_2 = period_index_2 + 1;
            last_adaptation_2 = 1;
            tau_2 = 0;
            t1 = t0;
            %disp ('Hello');
        end
    end
elseif ((Vxt > Vlth) && (current_period_2 > candidate_period(1)))
    if (last_adaptation_2 == 1)
        current_period_2 = candidate_period(period_index_2 - 1);
        period_index_2 = period_index_2 - 1;
        last_adaptation_2 = -1;
        tau_2 = 0;
        t1 = timer;
        Vxt0_1 = Vxt;
        %disp('Hi');
    elseif ((last_adaptation_2 == -1) && (Vxt > ((1 - (beta/alpha_2))^(timer-t0))*Vxt0_1))
        current_period_2 = candidate_period(period_index_2 - 1);
        period_index_2 = period_index_2 - 1;
        last_adaptation_2 = -1;
        t1 = timer;
        tau_2 = 0;
        %disp('Hey');
    end
else
    current_period_2 = candidate_period(period_index_2);
    %last_adaptation_2 = 0;
    tau_2 = 0;
    t1 = timer;
    %disp('HiHi');
end
%end   
y = current_period_2;
%disp(current_period_1);
Vxt0 = Vxt0_1;
end

== matlab function Control_Loop4_2Model/PeriodAdaptation_3 ==
  data: timer input; Vxt input; y output; period_index_3 data_store_memory; t0 input; t1 output; Vxt0_1 input; Vxt0 output; current_period_3 data_store_memory; tau_3 data_store_memory; last_adaptation_3 data_store_memory
function [y,t1,Vxt0]= fcn(timer,Vxt,t0,Vxt0_1)
%#codegen
global current_period_3;
global period_index_3;
global tau_3;
global last_adaptation_3;

t1 = 0;
candidate_period = [15,30,60];   
no_of_candidates = 3;
alpha_1 = -2.4439;
alpha_2 = 2.2439;
beta = 1;
X_SE2 = 0.01;
Lambda = 0.1;
Vlth = alpha_1*X_SE2;
Vdth = Vlth * Lambda;

%disp(Vxt);
%disp(Vdth);
if (Vxt < Vdth)
    tau_3 = tau_3 + 1; 
    disp(tau_3);
    if (tau_3 == 100)
        if (current_period_3 < candidate_period(no_of_candidates))
            current_period_3 = candidate_period(period_index_3 + 1);
            period_index_3 = period_index_3 + 1;
            last_adaptation_3 = 1;
            tau_3 = 0;
            t1 = t0;
            %disp ('Hello');
        end
    end
elseif ((Vxt > Vlth) && (current_period_3 > candidate_period(1)))
    if (last_adaptation_3 == 1)
        current_period_3 = candidate_period(period_index_3 - 1);
        period_index_3 = period_index_3 - 1;
        last_adaptation_3 = -1;
        tau_3 = 0;
        t1 = timer;
        Vxt0_1 = Vxt;
        %disp('Hi');
    elseif ((last_adaptation_3 == -1) && (Vxt > ((1 - (beta/alpha_2))^(timer-t0))*Vxt0_1))
        current_period_3 = candidate_period(period_index_3 - 1);
        period_index_3 = period_index_3 - 1;
        last_adaptation_3 = -1;
        t1 = timer;
        tau_3 = 0;
        %disp('Hey');
    end
else
    current_period_3 = candidate_period(period_index_3);
    %last_adaptation_3 = 0;
    tau_3 = 0;
    t1 = timer;
    %disp('HiHi');
end
%end   
y = current_period_3;
%disp(current_period_1);
Vxt0 = Vxt0_1;
end

== matlab function Control_Loop4_2Model/PeriodAdaptation_1 ==
  data: timer input; Vxt input; y output; period_index_1 data_store_memory; t0 input; t1 output; Vxt0_1 input; Vxt0 output; current_period_1 data_store_memory; tau_1 data_store_memory; last_adaptation_1 data_store_memory
function [y,t1,Vxt0]= fcn(timer,Vxt,t0,Vxt0_1)
%#codegen
global current_period_1;
global period_index_1;
global tau_1;
global last_adaptation_1;

t1 = 0;
candidate_period = [10,20,30,60];   
no_of_candidates = 3;
alpha_1 = -31.4772;
alpha_2 = 3.7059;
beta = 1;
X_SE2 = 0.01;
Lambda = 0.1;
Vlth = alpha_1*X_SE2;
Vdth = Vlth * Lambda;

disp (tau_1);
disp(Vxt);
disp(Vdth);
disp(Vlth)
if (Vxt < Vdth)
    tau_1 = tau_1 + 1; 
    if (tau_1 == 100)
        if (current_period_1 < candidate_period(no_of_candidates))
            current_period_1 = candidate_period(period_index_1 + 1);
            period_index_1 = period_index_1 + 1;
            last_adaptation_1 = 1;
            %la_1 = 1;
            tau_1 = 0;
            t1 = t0;
            disp ('Hello');
        end
    end
elseif ((Vxt > Vlth) && (current_period_1 > candidate_period(1)))
    disp('Inside Rate Increase');
    if (last_adaptation_1 == 1)
    %if (la_1 == 1)
        disp('Inside la_1');
        current_period_1 = candidate_period(period_index_1 - 1);
        period_index_1 = period_index_1 - 1;
        last_adaptation_1 = -1;
        %la_1 = -1;
        tau_1 = 0;
        t1 = timer;
        Vxt0_1 = Vxt;
        disp('Hi');
    elseif ((last_adaptation_1 == -1) && (Vxt > ((1 - (beta/alpha_2))^(timer-t0))*Vxt0_1))
    %if ((la_1 == -1) && (Vxt > ((1 - (beta/alpha_2))^(timer-t0))*Vxt0_1))
        current_period_1 = candidate_period(period_index_1 - 1);
        period_index_1 = period_index_1 - 1;
        last_adaptation_1 = -1;
        %la_1 = -1;
        t1 = timer;
        tau_1 = 0;
        disp('Hey');
    end
else
    current_period_1 = candidate_period(period_index_1);
    %last_adaptation_1 = 0;
    tau_1 = 0;
    t1 = timer;
    disp('HiHi');
end
%end   
disp(Vxt0_1);
y = current_period_1;
%disp(current_period_1);
Vxt0 = Vxt0_1;
%la_1 = last_adaptation_1;
end

== matlab function Control_Loop4_2Model/PeriodAdaptation_4 ==
  data: timer input; Vxt input; y output; period_index_4 data_store_memory; t0 input; t1 output; Vxt0_1 input; Vxt0 output; current_period_4 data_store_memory; tau_4 data_store_memory; last_adaptation_4 data_store_memory
function [y,t1,Vxt0]= fcn(timer,Vxt,t0,Vxt0_1)
%#codegen
global current_period_4;
global period_index_4;
global tau_4;
global last_adaptation_4;

t1 = 0;
candidate_period = [15,30,60];   
no_of_candidates = 3;
alpha_1 = -2.4439;
alpha_2 = 2.2439;
beta = 1;
X_SE2 = 0.01;
Lambda = 0.1;
Vlth = alpha_1*X_SE2;
Vdth = Vlth * Lambda;

%disp(tau_4);
%disp(Vxt);
%disp(Vdth);
%disp(Vlth);
if (Vxt < Vdth)
    tau_4 = tau_4 + 1; 
    %disp(tau_4);
    if (tau_4 == 100)
        if (current_period_4 < candidate_period(no_of_candidates))
            current_period_4 = candidate_period(period_index_4 + 1);
            period_index_4 = period_index_4 + 1;
            last_adaptation_4 = 1;
            tau_4 = 0;
            t1 = t0;
            %disp ('Hello');
        end
    end
elseif ((Vxt > Vlth) && (current_period_4 > candidate_period(1)))
    if (last_adaptation_4 == 1)
        current_period_4 = candidate_period(period_index_4 - 1);
        period_index_4 = period_index_4 - 1;
        last_adaptation_4 = -1;
        tau_4 = 0;
        t1 = timer;
        Vxt0_1 = Vxt;
        %disp('Hi');
    elseif ((last_adaptation_4 == -1) && (Vxt > ((1 - (beta/alpha_2))^(timer-t0))*Vxt0_1))
        current_period_4 = candidate_period(period_index_4 - 1);
        period_index_4 = period_index_4 - 1;
        last_adaptation_4 = -1;
        t1 = timer;
        tau_4 = 0;
        %disp('Hey');
    end
else
    current_period_4 = candidate_period(period_index_4);
    %last_adaptation_4 = 0;
    tau_4 = 0;
    t1 = timer;
    %disp('HiHi');
end
%end   
y = current_period_4;
%disp(current_period_1);
Vxt0 = Vxt0_1;
end

== matlab function Control_Loop4_2Model/combineDecimal_1 ==
  data: u1 input; u2 input; y output
function y = fcn(u1,u2)
y = 0;
if (u2 >= 2000 && u2 < 3000)
    u2 = u2 - 2000;
%#codegen
if (u1 >= 1000)
    u1 = u1 - 1000;
    %if (u2 >= 1000)
     %   u2 = u2 - 1000;
        y = - (u1 + u2*0.001);
        %y2 = y;
        %y1 = u1_prev;
    %else
     %   y = - (u1 + u2*0.001);
     %   y1 = y;
     %   y2 = u2_prev;
    %end
else
    %if (u2 >= 1000)
    %    u2 = u2 - 1000;
        y = (u1 + u2*0.001);
     %   y2 = y;
     %   y1 = u1_prev;
    %else
     %   y = (u1 + u2*0.001);
     %   y1 = y;
     %   y2 = u2_prev;
    %end
end
end
%x = y;
%x2 = y2;
%if (u1 > 2047)
%    u1 = -(4096 - u1);
%    u2 = u2 * (-0.01);
%else
%    u2 = u2 * (0.01);
%end
%y = u1 + u2;
%if y == 0.00
%    if x == 0.00
%        y = 0.00;
%    end
%end
%x1 = y;
%if u > 2047
  %  u = -(4096 - u);
%end
%u = u * 0.1;
%if u > 0.0
 %   y = u;
%elseif u < 0.0
%    y = u;
%else
%    y = x;
%end  
%if (u > 3095)
%    u = -(4096 - u)/10;
%else
%    u = u/10;
%end
%y = u;
%u = u/10 - 100;
%if (u > 0.0)
%    y = u;
%elseif (u < 0.0)
%    y = u;
%else
%if u == 0
%    y = x;
%else
%    y = u;
%end
end

== matlab function Control_Loop4_2Model/LowPowerBusInput ==
  data: y output; period_index_1 data_store_memory; period_index_2 data_store_memory; period_index_3 data_store_memory; period_index_4 data_store_memory
function y = fcn
%#codegen
global period_index_1;
global period_index_2;
global period_index_3;
global period_index_4;
%x1 = 0;
%x2 = 0;
%x3 = 0; 
%x4 = 0;
Period = [10 20 30 60;10 20 60 60;15 30 60 60;15 30 60 60];
    
%if (ne(current_period_1,BasePeriods(1)))
%    x1 = period_index_1;
%    BasePeriods(1) = Period(1,period_index_1);
%end
%if (ne(current_period_2,BasePeriods(2)))
%    x2 = period_index_2;
%    BasePeriods(2) = Period(2,period_index_2);
%end
%if (ne(current_period_3,BasePeriods(3)))
%    x3 = period_index_3;
%    BasePeriods(3) = Period(3,period_index_3);
%end
%if (ne(current_period_4,BasePeriods(4)))
%    x4 = period_index_4;
%    BasePeriods(4) = Period(4,period_index_4);
%end
y = 10^0 * (period_index_1 - 1) + 10^1 * (period_index_2 - 1) + 10^2 * (period_index_3 - 1) + 10^3 * (period_index_4 - 1);

end

== matlab function Control_Loop4_2Model/MATLAB Function ==
  data: y output; timer input
function y = fcn(timer)
%#codegen
%if timer >= 115 && timer < 135
%    y = 5;
%else
   y = 0;
%end
end
